simulink model "SLD_AC"  (R2023b)
settings: Solver=ode23tb  StartTime=0.0  StopTime=0.02  MaxStep=1e-4  RelTol=1e-3
undefined symbols (not defined in the file or in its folder): D1, Delta
libraries: spsCurrentMeasurementLib x3, spsParallelRLCLoadLib x3, spsVoltageMeasurementLib x3, spsThreePhaseParallelRLCLoadLib x2, spsThreePhaseTransformerTwoWindingsLib x1, spsThreePhaseSourceLib x1, spsThreePhasePISectionLineLib x1, spsThreePhaseVIMeasurementLib x1, spsThreePhaseBreakerLib x1, sps_lib x1
settings Model: Creator=HP  LastModifiedBy=HP

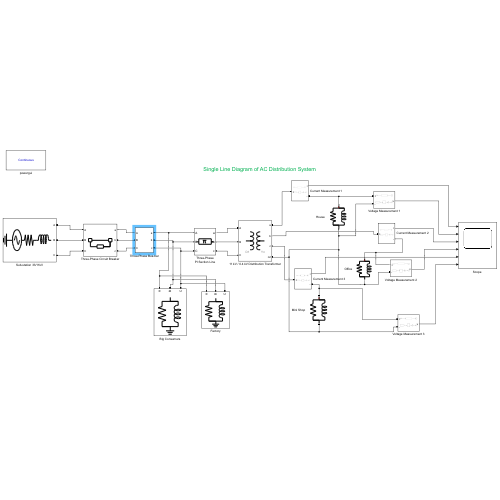
[thumbnail: Simulink's stored preview of the top-level diagram]
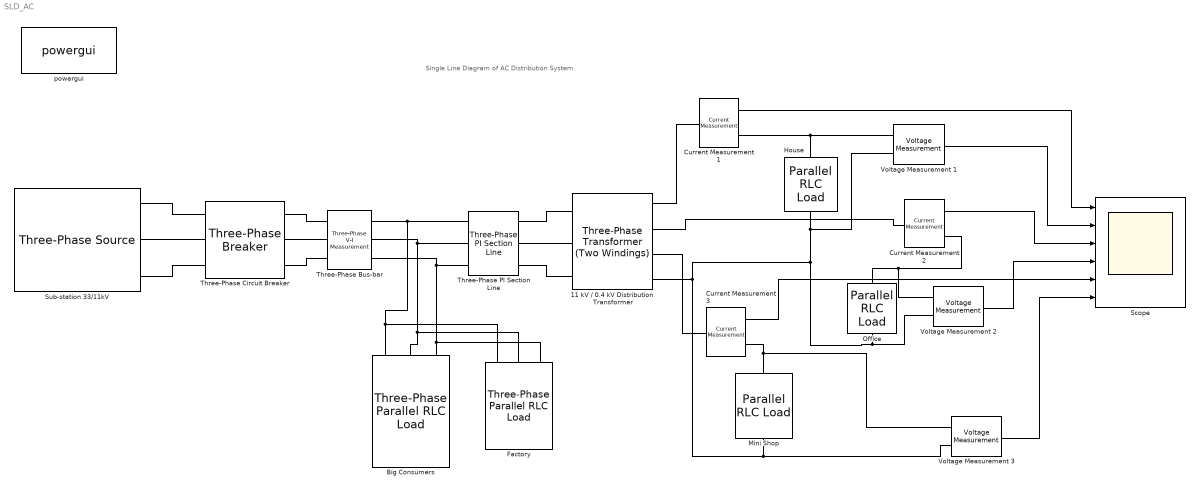
== system SLD_AC ==
  note: Single Line Diagram of AC Distribution System
  11 kV / 0.4 kV Distribution Transformer : spsThreePhaseTransformerTwoWindingsLib/Three-Phase Transformer (Two Windings)  Winding1Connection=Delta (D1)  Winding2Connection=Yn  CoreType=Three single-phase transformers  SetSaturation=off  Hysteresis=off  DataFile='hysteresis'  SetInitialFlux=off  Measurements=None  UNITS=pu  NominalPower=[ 250e6 , 60 ]  Winding1=[ 735e3 , 0.002 , 0.08 ]  Winding2=[ 315e3 , 0.002 , 0.08 ]  Rm=500  Lm=500  L0=0.5  Saturation=[ 0,0 ; 0.0024,1.2 ; 1.0,1.52 ]  InitialFluxes=[ 0.8 , -0.8 , 0.7 ]  BreakLoop=off  DiscreteSolver=Trapezoidal iterative  DataType=off  TransfoNumber=1
  Big Consumers : spsThreePhaseParallelRLCLoadLib/Three-Phase Parallel RLC Load  LConnTagsString=A|B|C  Configuration=Y (grounded)  NominalVoltage=11000  Vabc=[1e3 1e3 1e3]  Vabcp=[1e3 1e3 1e3]  NominalFrequency=50  UnbalancedPower=off  ActivePower=100000  InductivePower=48432  CapacitivePower=0  Pabc=[10e3 9e3 11e3]  QLabc=[100 90 110]  QCabc=[100 90 110]  Pabcp=[10e3 9e3 11e3]  QLabcp=[100 90 110]  QCabcp=[100 90 110]  Measurements=None  LoadType=constant Z
  Current Measurement 1 : spsCurrentMeasurementLib/Current Measurement  PhasorSimulation=off  OutputType=Complex  PSBequivalent=0
  Current Measurement 2 : spsCurrentMeasurementLib/Current Measurement  PhasorSimulation=off  OutputType=Complex  PSBequivalent=0
  Current Measurement 3 : spsCurrentMeasurementLib/Current Measurement  PhasorSimulation=off  OutputType=Complex  PSBequivalent=0
  Factory : spsThreePhaseParallelRLCLoadLib/Three-Phase Parallel RLC Load  LConnTagsString=A|B|C  Configuration=Y (grounded)  NominalVoltage=11000  Vabc=[1e3 1e3 1e3]  Vabcp=[1e3 1e3 1e3]  NominalFrequency=50  UnbalancedPower=off  ActivePower=500000  InductivePower=242161  CapacitivePower=0  Pabc=[10e3 9e3 11e3]  QLabc=[100 90 110]  QCabc=[100 90 110]  Pabcp=[10e3 9e3 11e3]  QLabcp=[100 90 110]  QCabcp=[100 90 110]  Measurements=None  LoadType=constant Z
  "House " : spsParallelRLCLoadLib/Parallel RLC Load  LConnTagsString=a  RConnTagsString=__new0  NominalVoltage=230  NominalFrequency=50  ActivePower=5e3  InductivePower=2420  CapacitivePower=0  Setx0=off  InitialVoltage=0  SetiL0=off  InitialCurrent=0  Measurements=None  LoadType=constant Z
      settings: AttributesFormatString=\n  LibrarySourceBlock=sps_lib/Passives/Parallel RLC Load
  Mini Shop : spsParallelRLCLoadLib/Parallel RLC Load  LConnTagsString=a  RConnTagsString=__new0  NominalVoltage=230  NominalFrequency=50  ActivePower=5e3  InductivePower=2420  CapacitivePower=0  Setx0=off  InitialVoltage=0  SetiL0=off  InitialCurrent=0  Measurements=None  LoadType=constant Z
      settings: AttributesFormatString=\n  LibrarySourceBlock=sps_lib/Passives/Parallel RLC Load
  Office : spsParallelRLCLoadLib/Parallel RLC Load  LConnTagsString=a  RConnTagsString=__new0  NominalVoltage=230  NominalFrequency=50  ActivePower=5e3  InductivePower=2420  CapacitivePower=0  Setx0=off  InitialVoltage=0  SetiL0=off  InitialCurrent=0  Measurements=None  LoadType=constant Z
      settings: AttributesFormatString=\n  LibrarySourceBlock=sps_lib/Passives/Parallel RLC Load
  "Scope " : Scope  NumInputPorts=6
  Sub-station 33/11kV : spsThreePhaseSourceLib/Three-Phase Source  InternalConnection=Yg  VoltagePhases=off  Voltage=33e3  PhaseAngle=0  Voltage_phases=[25e3 25e3 25e3]/sqrt(3)  PhaseAngles_phases=[0 -120 +120]  Frequency=50  NonIdealSource=on  SpecifyImpedance=off  Resistance=0.8929  Inductance=16.58e-3  ShortCircuitLevel=100e6  BaseVoltage=33e3  XRratio=7  BusType=swing  Pref=10e3  Qref=0  Prefabc=[10e3, 10e3, 10e3]  Qrefabc=[0, 0, 0]  Qmin=-inf  Qmax=inf
  Three-Phase PI Section Line : spsThreePhasePISectionLineLib/Three-Phase PI Section Line  LConnTagsString=a|b|c  RConnTagsString=A|B|C  Length=5  Frequency=50  Resistances=[ 0.20 1.2]  Inductances=[ 1.0e-3 3.5e-3]  Capacitances=[1.2e-8 2.5e-9]
  Three-Phase Bus-bar : spsThreePhaseVIMeasurementLib/Three-Phase V-I Measurement  VoltageMeasurement=no  SetLabelV=off  LabelV=Vabc  Vpu=off  VpuLL=off  CurrentMeasurement=no  SetLabelI=off  LabelI=Iabc  Ipu=off  Pbase=100e6  Vbase=500e3  OutputType=Complex  PhasorSimulation=off  PSBequivalent=0
  Three-Phase Circuit Breaker : spsThreePhaseBreakerLib/Three-Phase Breaker  InitialState=closed  SwitchA=on  SwitchB=on  SwitchC=on  SwitchTimes=[1/50 0.1]  External=off  BreakerResistance=0.01  SnubberResistance=1e6  SnubberCapacitance=inf  Measurements=None
  Voltage Measurement 1 : spsVoltageMeasurementLib/Voltage Measurement  PhasorSimulation=off  OutputType=Complex  PSBequivalent=0
  Voltage Measurement 2 : spsVoltageMeasurementLib/Voltage Measurement  PhasorSimulation=off  OutputType=Complex  PSBequivalent=0
  Voltage Measurement 3 : spsVoltageMeasurementLib/Voltage Measurement  PhasorSimulation=off  OutputType=Complex  PSBequivalent=0
  powergui : sps_lib/powergui  Priority=1  SimulationMode=Continuous  SampleTime=50e-6  frequency=60  Iterations=50  frequencyindice=50  Pbase=100e6  ErrMax=1e-4  UnitsV=kV  UnitsW=MW  buscounter=0  FunctionMessages=off  echomessages=off  EnableUseOfTLC=off  CurrentSourceSwitches=off  DisableSnubberDevices=off  DisableRonSwitches=off  DisableVfSwitches=off  DisplayEquations=off  AutomaticDiscreteSolvers=off  SolverType=Tustin/Backward Euler (TBE)  Interpol=off  ExternalGateDelay=off  methode=off  Ts=100  x0status=blocks  SPID=on  SwTol=0  HookPort=off  NonlinearTolerance=1e-4  nMaxIteration=100  ContinueOnMaxIteration=off  RestoreLinks=warning  ResistiveCurrentMeasurement=off  Frange=[0:2:500]  Ylog=off  Xlog=on  ShowGrid=off  save=off  variable=ZData  structure=0  ZoomFFT=off  StartTime=0.0  cycles=1  DisplayStyle=1  fundamental=60  FreqAxis=off  MaxFrequency=1000  frequencyindicesteady=1  RmsSteady=1  display=off
  wires:
  Voltage Measurement 1/1 -> "Scope "/2
  Current Measurement 1/1 -> "Scope "/1
  Current Measurement 2/1 -> "Scope "/3
  Voltage Measurement 2/1 -> "Scope "/4
  Current Measurement 3/1 -> "Scope "/5
  Voltage Measurement 3/1 -> "Scope "/6
  connections:
  Sub-station 33/11kV/RConn1 -- Three-Phase Circuit Breaker/LConn1
  Three-Phase Circuit Breaker/LConn2 -- Sub-station 33/11kV/RConn2
  Sub-station 33/11kV/RConn3 -- Three-Phase Circuit Breaker/LConn3
  Three-Phase Bus-bar/LConn1 -- Three-Phase Circuit Breaker/RConn1
  Three-Phase Circuit Breaker/RConn2 -- Three-Phase Bus-bar/LConn2
  Three-Phase Circuit Breaker/RConn3 -- Three-Phase Bus-bar/LConn3
  Three-Phase PI Section Line/LConn1 -- Factory/LConn1 -- Big Consumers/LConn1 -- Three-Phase Bus-bar/RConn1
  Three-Phase PI Section Line/LConn2 -- Three-Phase Bus-bar/RConn2 -- Factory/LConn2 -- Big Consumers/LConn2
  Three-Phase Bus-bar/RConn3 -- Factory/LConn3 -- Big Consumers/LConn3 -- Three-Phase PI Section Line/LConn3
  11 kV / 0.4 kV Distribution Transformer/LConn2 -- Three-Phase PI Section Line/RConn2
  Three-Phase PI Section Line/RConn3 -- 11 kV / 0.4 kV Distribution Transformer/LConn3
  Three-Phase PI Section Line/RConn1 -- 11 kV / 0.4 kV Distribution Transformer/LConn1
  "House "/LConn1 -- Current Measurement 1/RConn1 -- Voltage Measurement 1/LConn1
  Office/LConn1 -- Current Measurement 2/RConn1 -- Voltage Measurement 2/LConn1
  "House "/RConn1 -- Voltage Measurement 2/LConn2 -- Office/RConn1 -- Mini Shop/RConn1 -- Voltage Measurement 3/LConn2 -- 11 kV / 0.4 kV Distribution Transformer/RConn4 -- Voltage Measurement 1/LConn2
  Mini Shop/LConn1 -- Current Measurement 3/RConn1 -- Voltage Measurement 3/LConn1
  11 kV / 0.4 kV Distribution Transformer/RConn1 -- Current Measurement 1/LConn1
  Current Measurement 2/LConn1 -- 11 kV / 0.4 kV Distribution Transformer/RConn2
  11 kV / 0.4 kV Distribution Transformer/RConn3 -- Current Measurement 3/LConn1
